simulink model "motortest2013"  (Simulink 7.3)
settings: Solver=FixedStepDiscrete  StartTime=0.0  StopTime=inf  FixedStep=1  MaxStep=0.2  RelTol=1e-3
undefined symbols (not defined in the file): RPM1, RPM2
settings Model: Creator=gclayton  LastModifiedBy=wildcat  SimulationMode=external
settings DebuggingCC: InheritedTsInSrcMsg=none
settings RTWCC: SystemTargetFile=rlnx.tlc  GenCodeOnly=on  TemplateMakefile=rlnx_ubuntu.tmf  Description=Linux Real-Time Target  ProcessScript=rlnx_make_rtw_hook
settings RTWCC: CustomInclude=|
  | /usr/local/include/opencv/
  | /usr/local/include/
settings CodeAppCC: GenerateComments=off  SimulinkBlockComments=off
settings STFCustomTargetCC: ModelReferenceCompliant=off  MatFileLogging=on  SystemTargetFile=rlnx.tlc
settings GRTTargetCC: ModelReferenceCompliant=off  ParMdlRefBuildCompliant=off  CompOptLevelCompliant=off  ExtMode=on  ExtModeMexArgs='10.0.0.2'
settings CustomProperty: DataType=string  Value=-lm -ldl /usr/local/lib/libopencv_highgui.so.2.4
settings EnumStrPairs: String=PC

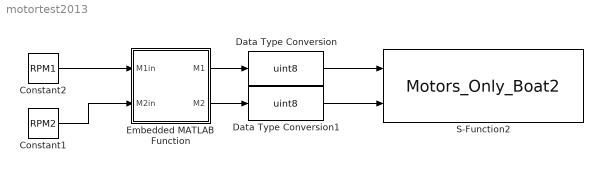
== system motortest2013 ==
  Constant1 : Constant  Value=RPM2
  Constant2 : Constant  Value=RPM1
  Data Type Conversion : DataTypeConversion  OutDataTypeMode=uint8  OutDataTypeStr=uint8
  Data Type Conversion1 : DataTypeConversion  OutDataTypeMode=uint8  OutDataTypeStr=uint8
  Embedded MATLAB Function : Stateflow chart  TreatAsAtomicUnit=on
  S-Function2 : S-Function  FunctionName=Motors_Only_Boat2  EnableBusSupport=off
  wires:
  Embedded MATLAB Function/1(M1) -> Data Type Conversion/1
  Embedded MATLAB Function/2(M2) -> Data Type Conversion1/1
  Data Type Conversion/1 -> S-Function2/1
  Data Type Conversion1/1 -> S-Function2/2
  Constant2/1 -> Embedded MATLAB Function/1(M1in)
  Constant1/1 -> Embedded MATLAB Function/2(M2in)

== matlab function Embedded MATLAB Function ==
  data: M1in input double; M1 output double; M2in input double; M2 output double
function [M1, M2] = MotorPackets(M1in, M2in)
%#eml

M1 = 0;
M2 = 1;

if M1in <= 0
    M1 = M1+2;
end

if M2in <= 0
    M2 = M2+2;
end

M1 = M1 + round(abs(M1in)*0.1)*4;
M2 = M2 + round(abs(M2in)*0.1)*4;
